simulink model "Modes-Toggling"  (R2021b)
settings: Solver=FixedStepAuto  StartTime=0.0  StopTime=10.0  RelTol=1e-3  EnableMultiTasking=on
libraries: legoev3lib x3, simulink x2, simulink_extras x2
settings Model: ExtModeTrigDuration=2  Creator=s142  LastModifiedBy=s142
settings SolverCC: PositivePriorityOrder=on
settings OptimizationCC: EnhancedBackFolding=on  PassReuseOutputArgsAs=Individual arguments  ZeroExternalMemoryAtStartup=off  ZeroInternalMemoryAtStartup=off  MaxStackSize=64  OptimizeBlockOrder=speed  DifferentSizesBufferReuse=on  OptimizationCustomize=off  EfficientTunableParamExpr=on
settings DebuggingCC: ParameterTunabilityLossMsg=error
settings HardwareCC: ProdBitPerPointer=32  ProdBitPerSizeT=32  ProdBitPerPtrDiffT=32  ProdLargestAtomicInteger=Long  ProdWordSize=32  ProdHWDeviceType=ARM Compatible->ARM 9
settings SFSimCC: MATLABDynamicMemAlloc=off
settings RTWCC: Description=Embedded Coder  SystemTargetFile=ert.tlc  HardwareBoard=LEGO MINDSTORMS EV3  TLCOptions="-aInlineSetEventsForThisBaseRateFcn=TLC_FALSE -aSuppressMultiTaskScheduler=TLC_FALSE  -aRateBasedStepFcn=0"  TemplateMakefile=ert_default_tmf  Toolchain=Sourcery G++ Lite v2009q3
settings CodeAppCC: ForceParamTrailComments=on  IgnoreCustomStorageClasses=off  OperatorAnnotations=on  SimulinkDataObjDesc=on  SFDataObjDesc=on  InsertBlockDesc=on
settings ERTTargetCC: SupportContinuousTime=on  SupportVariableSizeSignals=on  ExtModeTransport=2  ExtModeStaticAlloc=on  ExtModeMexFile=ext_xcp  ExtModeIntrfLevel=Level2 - Open

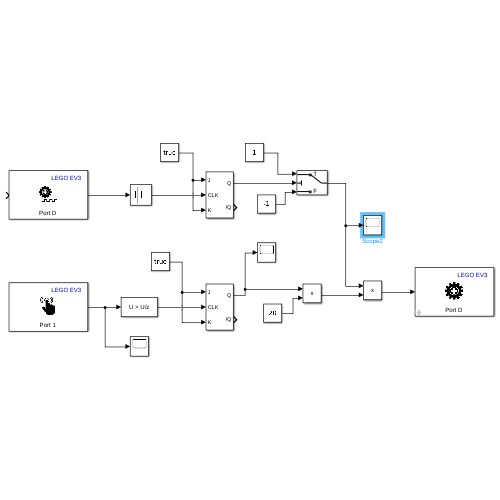
[thumbnail: Simulink's stored preview of the top-level diagram]
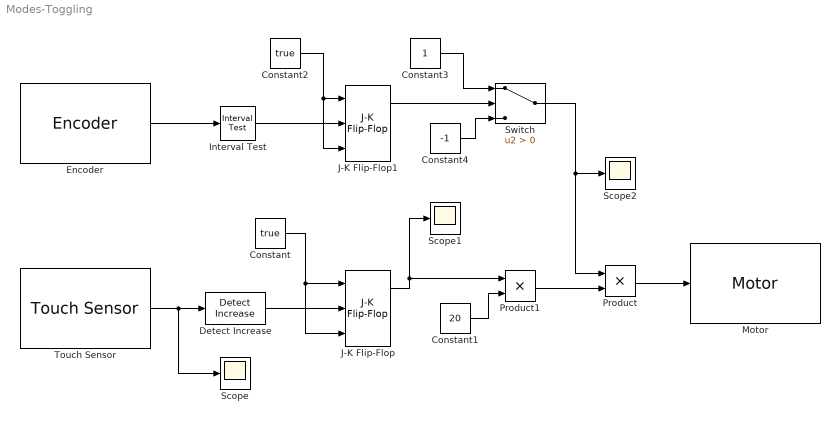
== system Modes-Toggling ==
  Constant : Constant  Value=true  OutDataTypeStr=boolean
  Constant1 : Constant  Value=20
  Constant2 : Constant  Value=true  OutDataTypeStr=boolean
  Constant3 : Constant
  Constant4 : Constant  Value=-1
  Detect Increase : simulink/Logic and Bit Operations/Detect Increase  vinit=0.0  OutDataTypeStr=boolean
  Encoder : legoev3lib/Encoder  portNumber=D  opMode=Reset by external signal  sampleTime=0.1
      settings: SourceProductBaseCode=LEGOEV3
  Interval Test : simulink/Logic and Bit Operations/Interval Test  IntervalClosedRight=on  uplimit=60  IntervalClosedLeft=on  lowlimit=-60  OutDataTypeStr=boolean
  J-K Flip-Flop : simulink_extras/Flip Flops/J-K Flip-Flop  initial_condition=0
  J-K Flip-Flop1 : simulink_extras/Flip Flops/J-K Flip-Flop  initial_condition=0
  Motor : legoev3lib/Motor  sportNumber=D  sstopAction=Brake
  Product : Product
  Product1 : Product
  Scope : Scope
  Scope1 : Scope
  Scope2 : Scope
  Switch : Switch  Criteria=u2 > Threshold
  Touch Sensor : legoev3lib/Touch Sensor  portNumber=1  sampleTime=0.1
      settings: SourceProductBaseCode=LEGOEV3
  wires:
  Touch Sensor/1 -> Detect Increase/1, Scope/1
  Detect Increase/1 -> J-K Flip-Flop/2
  Constant/1 -> J-K Flip-Flop/1, J-K Flip-Flop/3
  J-K Flip-Flop/1 -> Product1/1, Scope1/1
  Product/1 -> Motor/1
  Constant2/1 -> J-K Flip-Flop1/3, J-K Flip-Flop1/1
  J-K Flip-Flop1/1 -> Switch/2
  Constant4/1 -> Switch/3
  Constant3/1 -> Switch/1
  Switch/1 -> Product/1, Scope2/1
  Encoder/1 -> Interval Test/1
  Interval Test/1 -> J-K Flip-Flop1/2
  Constant1/1 -> Product1/2
  Product1/1 -> Product/2
